simulink model "AutonomousModel_V3"  (R2020b)
settings: Solver=ode23t  StartTime=0.0  StopTime=180.1  FixedStep=0.05  RelTol=1e-3  EnableMultiTasking=on
model workspace (MAT data in the model file):
  mapForSim : object (value not decoded)
  occGrid : robotics.BinaryOccupancyGrid (value not decoded)
undefined symbols (not defined in the file): cellLevel, cellPose, cellTypeArray, FloorSurface, isoPoses, platformPoses, PlowSurface, Ref, RobotSurface, WallSurface, X, Y, Z
libraries: sm_lib x286, nesl_utility x157, simulink x72, pid_lib x3
(part 2 of 14)

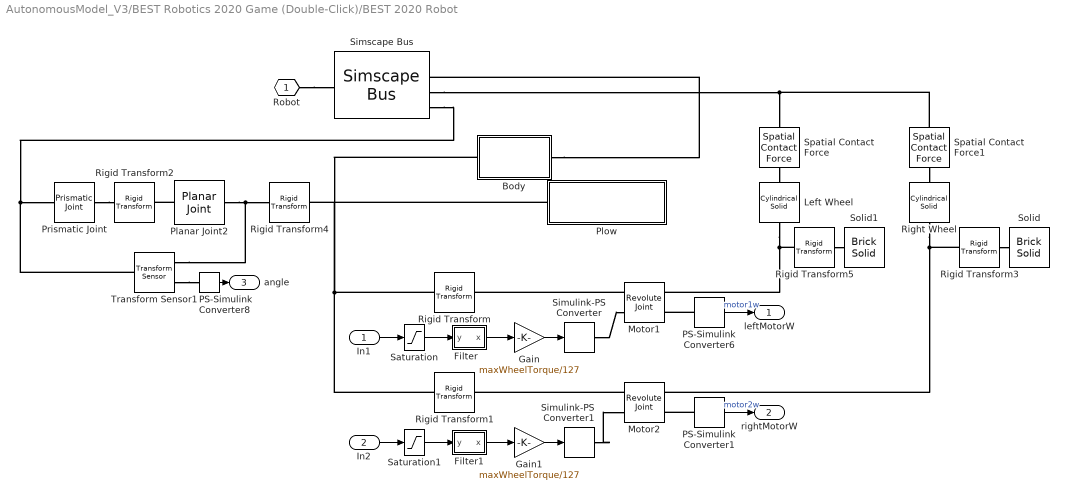
== system AutonomousModel_V3/BEST Robotics 2020 Game (Double-Click)/BEST 2020 Robot ==
  In1 : Inport
  In2 : Inport  Port=2
  Body : Subsystem
  Filter : Subsystem
  Filter1 : Subsystem
  Gain : Gain  Gain=maxWheelTorque/127
  Gain1 : Gain  Gain=maxWheelTorque/127
  Left Wheel : sm_lib/Body Elements/Cylindrical Solid  GraphicAmbientColor=[0.15 0.15 0.15 1.0]  BasedOnType=Mass  CenterOfMass=[0 0 0]  CenterOfMassUnits=m  GraphicDiffuseColor=wheelColor  CylinderLength=wheelThickness  CylinderLengthUnits=m  CylinderRadius=wheelRadius  CylinderRadiusUnits=m  Density=1000  DensityUnits=kg/m^3  DoExposeReferenceFrame=on  GraphicEmissiveColor=[0.0 0.0 0.0 1.0]  ExportEntireGeometry=on  SerializedFrames=<Frames/>  MarkerShape=Sphere  MarkerSize=10  GraphicType=FromGeometry  InertiaType=CalculateFromGeometry  Mass=wheelMass  MassUnits=kg  MomentsOfInertia=[1 1 1]  MomentsOfInertiaUnits=kg*m^2  GraphicOpacity=1.0  ProductsOfInertia=[1 1 1]  ProductsOfInertiaUnits=kg*m^2  GraphicShininess=75  GraphicSpecularColor=[0.5 0.5 0.5 1.0]  GraphicVisPropType=SimpleVisualProperties
  Motor1 : sm_lib/Joints/Revolute Joint  JointMode=Normal  SenseConstraintForce=off  SenseConstraintForceX=off  SenseConstraintForceY=off  SenseConstraintForceZ=off  SenseConstraintTorque=off  SenseConstraintTorqueX=off  SenseConstraintTorqueY=off  SenseConstraintTorqueZ=off  SenseTotalForce=off  SenseTotalForceX=off  SenseTotalForceY=off  SenseTotalForceZ=off  SenseTotalTorque=off  SenseTotalTorqueX=off  SenseTotalTorqueY=off  SenseTotalTorqueZ=off  CompositeWrenchDir=FollowerOnBase  CompositeWrenchFrame=BaseFrame  EquilibriumPosition=0  EquilibriumPositionUnits=deg  SpringStiffness=0  SpringStiffnessUnits=N*m/deg  DampingCoefficient=0.004  DampingCoefficientUnits=N*m/(deg/s)  TorqueActuationMode=InputTorque  MotionActuationMode=ComputedMotion  SensePosition=off  SenseVelocity=on  SenseAcceleration=off  SenseTorqueForce=off  SenseLowerLimitTorqueForce=off  SenseUpperLimitTorqueForce=off  LowerLimitSpecify=off  LowerLimitBound=-90  LowerLimitBoundUnits=deg  LowerLimitStiffness=1e4  LowerLimitStiffnessUnits=N*m/deg  LowerLimitDamping=10  LowerLimitDampingUnits=N*m/(deg/s)  LowerLimitTransitionRegionWidth=0.1  LowerLimitTransitionRegionWidthUnits=deg  UpperLimitSpecify=off  UpperLimitBound=90  UpperLimitBoundUnits=deg  UpperLimitStiffness=1e4  UpperLimitStiffnessUnits=N*m/deg  UpperLimitDamping=10  UpperLimitDampingUnits=N*m/(deg/s)  UpperLimitTransitionRegionWidth=0.1  UpperLimitTransitionRegionWidthUnits=deg  PositionTargetSpecify=off  PositionTargetPriority=High  PositionTargetValue=0  PositionTargetValueUnits=deg  VelocityTargetSpecify=off  VelocityTargetPriority=High  VelocityTargetValue=0  VelocityTargetValueUnits=deg/s
  Motor2 : sm_lib/Joints/Revolute Joint  JointMode=Normal  SenseConstraintForce=off  SenseConstraintForceX=off  SenseConstraintForceY=off  SenseConstraintForceZ=off  SenseConstraintTorque=off  SenseConstraintTorqueX=off  SenseConstraintTorqueY=off  SenseConstraintTorqueZ=off  SenseTotalForce=off  SenseTotalForceX=off  SenseTotalForceY=off  SenseTotalForceZ=off  SenseTotalTorque=off  SenseTotalTorqueX=off  SenseTotalTorqueY=off  SenseTotalTorqueZ=off  CompositeWrenchDir=FollowerOnBase  CompositeWrenchFrame=BaseFrame  EquilibriumPosition=0  EquilibriumPositionUnits=deg  SpringStiffness=0  SpringStiffnessUnits=N*m/deg  DampingCoefficient=0.004  DampingCoefficientUnits=N*m/(deg/s)  TorqueActuationMode=InputTorque  MotionActuationMode=ComputedMotion  SensePosition=off  SenseVelocity=on  SenseAcceleration=off  SenseTorqueForce=off  SenseLowerLimitTorqueForce=off  SenseUpperLimitTorqueForce=off  LowerLimitSpecify=off  LowerLimitBound=-90  LowerLimitBoundUnits=deg  LowerLimitStiffness=1e4  LowerLimitStiffnessUnits=N*m/deg  LowerLimitDamping=10  LowerLimitDampingUnits=N*m/(deg/s)  LowerLimitTransitionRegionWidth=0.1  LowerLimitTransitionRegionWidthUnits=deg  UpperLimitSpecify=off  UpperLimitBound=90  UpperLimitBoundUnits=deg  UpperLimitStiffness=1e4  UpperLimitStiffnessUnits=N*m/deg  UpperLimitDamping=10  UpperLimitDampingUnits=N*m/(deg/s)  UpperLimitTransitionRegionWidth=0.1  UpperLimitTransitionRegionWidthUnits=deg  PositionTargetSpecify=off  PositionTargetPriority=High  PositionTargetValue=0  PositionTargetValueUnits=deg  VelocityTargetSpecify=off  VelocityTargetPriority=High  VelocityTargetValue=0  VelocityTargetValueUnits=deg/s
  PS-Simulink Converter1 : nesl_utility/PS-Simulink Converter  PhysicalDomain=network_engine_domain  SubClassName=ps_output  LeftPortType=input  RightPortType=output  PseudoPeriodic=off  Frequencies=[]  Unit=1  AffineConversion=off
  PS-Simulink Converter6 : nesl_utility/PS-Simulink Converter  PhysicalDomain=network_engine_domain  SubClassName=ps_output  LeftPortType=input  RightPortType=output  PseudoPeriodic=off  Frequencies=[]  Unit=1  AffineConversion=off
  PS-Simulink Converter8 : nesl_utility/PS-Simulink Converter  PhysicalDomain=network_engine_domain  SubClassName=ps_output  LeftPortType=input  RightPortType=output  PseudoPeriodic=off  Frequencies=[]  Unit=deg  AffineConversion=off
  Planar Joint2 : sm_lib/Joints/Planar Joint  JointMode=Normal  SenseConstraintForce=off  SenseConstraintForceX=off  SenseConstraintForceY=off  SenseConstraintForceZ=off  SenseConstraintTorque=off  SenseConstraintTorqueX=off  SenseConstraintTorqueY=off  SenseConstraintTorqueZ=off  SenseTotalForce=off  SenseTotalForceX=off  SenseTotalForceY=off  SenseTotalForceZ=off  SenseTotalTorque=off  SenseTotalTorqueX=off  SenseTotalTorqueY=off  SenseTotalTorqueZ=off  CompositeWrenchDir=FollowerOnBase  CompositeWrenchFrame=BaseFrame  PxEquilibriumPosition=0  PxEquilibriumPositionUnits=m  PxSpringStiffness=0  PxSpringStiffnessUnits=N/m  PxDampingCoefficient=0  PxDampingCoefficientUnits=N/(m/s)  PxTorqueActuationMode=NoTorque  PxMotionActuationMode=ComputedMotion  PxSensePosition=off  PxSenseVelocity=off  PxSenseAcceleration=off  PxSenseTorqueForce=off  PxSenseLowerLimitTorqueForce=off  PxSenseUpperLimitTorqueForce=off  PxLowerLimitSpecify=off  PxLowerLimitBound=-1  PxLowerLimitBoundUnits=m  PxLowerLimitStiffness=1e6  PxLowerLimitStiffnessUnits=N/m  PxLowerLimitDamping=1e3  PxLowerLimitDampingUnits=N/(m/s)  PxLowerLimitTransitionRegionWidth=1e-4  PxLowerLimitTransitionRegionWidthUnits=m  PxUpperLimitSpecify=off  PxUpperLimitBound=1  PxUpperLimitBoundUnits=m  PxUpperLimitStiffness=1e6  PxUpperLimitStiffnessUnits=N/m  PxUpperLimitDamping=1e3  PxUpperLimitDampingUnits=N/(m/s)  PxUpperLimitTransitionRegionWidth=1e-4  PxUpperLimitTransitionRegionWidthUnits=m  PxPositionTargetSpecify=on  PxPositionTargetPriority=High  PxPositionTargetValue=startPose(1)  PxPositionTargetValueUnits=m  PxVelocityTargetSpecify=off  PxVelocityTargetPriority=High  PxVelocityTargetValue=0  PxVelocityTargetValueUnits=m/s  PyEquilibriumPosition=0  PyEquilibriumPositionUnits=m  PySpringStiffness=0  PySpringStiffnessUnits=N/m  PyDampingCoefficient=0  PyDampingCoefficientUnits=N/(m/s)  PyTorqueActuationMode=NoTorque  PyMotionActuationMode=ComputedMotion  PySensePosition=off  PySenseVelocity=off  PySenseAcceleration=off  PySenseTorqueForce=off  PySenseLowerLimitTorqueForce=off  PySenseUpperLimitTorqueForce=off  PyLowerLimitSpecify=off  PyLowerLimitBound=-1  PyLowerLimitBoundUnits=m  PyLowerLimitStiffness=1e6  PyLowerLimitStiffnessUnits=N/m  PyLowerLimitDamping=1e3  PyLowerLimitDampingUnits=N/(m/s)  PyLowerLimitTransitionRegionWidth=1e-4  PyLowerLimitTransitionRegionWidthUnits=m  PyUpperLimitSpecify=off  PyUpperLimitBound=1  PyUpperLimitBoundUnits=m  PyUpperLimitStiffness=1e6  PyUpperLimitStiffnessUnits=N/m  PyUpperLimitDamping=1e3  PyUpperLimitDampingUnits=N/(m/s)  PyUpperLimitTransitionRegionWidth=1e-4  PyUpperLimitTransitionRegionWidthUnits=m  PyPositionTargetSpecify=on  PyPositionTargetPriority=High  PyPositionTargetValue=startPose(2)  PyPositionTargetValueUnits=m  PyVelocityTargetSpecify=off  PyVelocityTargetPriority=High  PyVelocityTargetValue=0  PyVelocityTargetValueUnits=m/s  RzEquilibriumPosition=0  RzEquilibriumPositionUnits=deg  RzSpringStiffness=0  RzSpringStiffnessUnits=N*m/deg  RzDampingCoefficient=0  RzDampingCoefficientUnits=N*m/(deg/s)  RzTorqueActuationMode=NoTorque  RzMotionActuationMode=ComputedMotion  RzSensePosition=off  RzSenseVelocity=off  RzSenseAcceleration=off  RzSenseTorqueForce=off  RzSenseLowerLimitTorqueForce=off  RzSenseUpperLimitTorqueForce=off  RzLowerLimitSpecify=off  RzLowerLimitBound=-90  RzLowerLimitBoundUnits=deg  RzLowerLimitStiffness=1e4  RzLowerLimitStiffnessUnits=N*m/deg  RzLowerLimitDamping=10  RzLowerLimitDampingUnits=N*m/(deg/s)  RzLowerLimitTransitionRegionWidth=0.1  RzLowerLimitTransitionRegionWidthUnits=deg  RzUpperLimitSpecify=off  RzUpperLimitBound=90  RzUpperLimitBoundUnits=deg  RzUpperLimitStiffness=1e4  RzUpperLimitStiffnessUnits=N*m/deg  RzUpperLimitDamping=10  RzUpperLimitDampingUnits=N*m/(deg/s)  RzUpperLimitTransitionRegionWidth=0.1  RzUpperLimitTransitionRegionWidthUnits=deg  RzPositionTargetSpecify=off  RzPositionTargetPriority=High  RzPositionTargetValue=0  RzPositionTargetValueUnits=deg  RzVelocityTargetSpecify=off  RzVelocityTargetPriority=High  RzVelocityTargetValue=0  RzVelocityTargetValueUnits=deg/s
  Plow : Subsystem
  Prismatic Joint : sm_lib/Joints/Prismatic Joint  JointMode=Normal  SenseConstraintForce=off  SenseConstraintForceX=off  SenseConstraintForceY=off  SenseConstraintForceZ=off  SenseConstraintTorque=off  SenseConstraintTorqueX=off  SenseConstraintTorqueY=off  SenseConstraintTorqueZ=off  SenseTotalForce=off  SenseTotalForceX=off  SenseTotalForceY=off  SenseTotalForceZ=off  SenseTotalTorque=off  SenseTotalTorqueX=off  SenseTotalTorqueY=off  SenseTotalTorqueZ=off  CompositeWrenchDir=FollowerOnBase  CompositeWrenchFrame=BaseFrame  EquilibriumPosition=0  EquilibriumPositionUnits=m  SpringStiffness=0  SpringStiffnessUnits=N/m  DampingCoefficient=0  DampingCoefficientUnits=N/(m/s)  TorqueActuationMode=NoTorque  MotionActuationMode=ComputedMotion  SensePosition=off  SenseVelocity=off  SenseAcceleration=off  SenseTorqueForce=off  SenseLowerLimitTorqueForce=off  SenseUpperLimitTorqueForce=off  LowerLimitSpecify=off  LowerLimitBound=-1  LowerLimitBoundUnits=m  LowerLimitStiffness=1e6  LowerLimitStiffnessUnits=N/m  LowerLimitDamping=1e3  LowerLimitDampingUnits=N/(m/s)  LowerLimitTransitionRegionWidth=1e-4  LowerLimitTransitionRegionWidthUnits=m  UpperLimitSpecify=off  UpperLimitBound=1  UpperLimitBoundUnits=m  UpperLimitStiffness=1e6  UpperLimitStiffnessUnits=N/m  UpperLimitDamping=1e3  UpperLimitDampingUnits=N/(m/s)  UpperLimitTransitionRegionWidth=1e-4  UpperLimitTransitionRegionWidthUnits=m  PositionTargetSpecify=on  PositionTargetPriority=High  PositionTargetValue=0.02  PositionTargetValueUnits=m  VelocityTargetSpecify=off  VelocityTargetPriority=High  VelocityTargetValue=0  VelocityTargetValueUnits=m/s
  Right Wheel : sm_lib/Body Elements/Cylindrical Solid  GraphicAmbientColor=[0.15 0.15 0.15 1.0]  BasedOnType=Mass  CenterOfMass=[0 0 0]  CenterOfMassUnits=m  GraphicDiffuseColor=wheelColor  CylinderLength=wheelThickness  CylinderLengthUnits=m  CylinderRadius=wheelRadius  CylinderRadiusUnits=m  Density=1000  DensityUnits=kg/m^3  DoExposeReferenceFrame=on  GraphicEmissiveColor=[0.0 0.0 0.0 1.0]  ExportEntireGeometry=on  SerializedFrames=<Frames/>  MarkerShape=Sphere  MarkerSize=10  GraphicType=FromGeometry  InertiaType=CalculateFromGeometry  Mass=wheelMass  MassUnits=kg  MomentsOfInertia=[1 1 1]  MomentsOfInertiaUnits=kg*m^2  GraphicOpacity=1.0  ProductsOfInertia=[1 1 1]  ProductsOfInertiaUnits=kg*m^2  GraphicShininess=75  GraphicSpecularColor=[0.5 0.5 0.5 1.0]  GraphicVisPropType=SimpleVisualProperties
  Rigid Transform : sm_lib/Frames and Transforms/Rigid Transform  TranslationMethod=StandardAxis  TranslationStandardOffset=wheelBase/2  TranslationLengthUnit=m  TranslationStandardAxis=+Y  TranslationCartesianOffset=[0 0 0]  TranslationROffset=0  TranslationROffsetUnits=m  TranslationZOffset=0  TranslationZOffsetUnits=m  TranslationThetaOffset=0  TranslationThetaOffsetUnits=deg  RotationMethod=AlignedAxes  RotationAngleUnits=deg  RotationStandardAxis=+Z  RotationAngle=0.0  RotationArbitraryAxis=[0 0 1]  FollAlignAxisA=+Z  BaseAlignAxisA=+Y  FollAlignAxisB=+X  BaseAlignAxisB=+X  RotationSequenceAxes=FollowerAxes  RotationSequence=XYX  RotationSequenceAngles=[0 0 0]  RotationSequenceAnglesUnits=deg  RotationMatrix=[1 0 0; 0 1 0; 0 0 1]
  Rigid Transform1 : sm_lib/Frames and Transforms/Rigid Transform  TranslationMethod=StandardAxis  TranslationStandardOffset=wheelBase/2  TranslationLengthUnit=m  TranslationStandardAxis=-Y  TranslationCartesianOffset=[0 0 0]  TranslationROffset=0  TranslationROffsetUnits=m  TranslationZOffset=0  TranslationZOffsetUnits=m  TranslationThetaOffset=0  TranslationThetaOffsetUnits=deg  RotationMethod=AlignedAxes  RotationAngleUnits=deg  RotationStandardAxis=+Z  RotationAngle=0.0  RotationArbitraryAxis=[0 0 1]  FollAlignAxisA=+Z  BaseAlignAxisA=+Y  FollAlignAxisB=+X  BaseAlignAxisB=+X  RotationSequenceAxes=FollowerAxes  RotationSequence=XYX  RotationSequenceAngles=[0 0 0]  RotationSequenceAnglesUnits=deg  RotationMatrix=[1 0 0; 0 1 0; 0 0 1]
  Rigid Transform2 : sm_lib/Frames and Transforms/Rigid Transform  TranslationMethod=StandardAxis  TranslationStandardOffset=wheelRadius  TranslationLengthUnit=m  TranslationStandardAxis=+Z  TranslationCartesianOffset=[0 0 0]  TranslationROffset=0  TranslationROffsetUnits=m  TranslationZOffset=0  TranslationZOffsetUnits=m  TranslationThetaOffset=0  TranslationThetaOffsetUnits=deg  RotationMethod=None  RotationAngleUnits=deg  RotationStandardAxis=+Z  RotationAngle=0.0  RotationArbitraryAxis=[0 0 1]  FollAlignAxisA=+Z  BaseAlignAxisA=+Y  FollAlignAxisB=+X  BaseAlignAxisB=+X  RotationSequenceAxes=FollowerAxes  RotationSequence=XYX  RotationSequenceAngles=[0 0 0]  RotationSequenceAnglesUnits=deg  RotationMatrix=[1 0 0; 0 1 0; 0 0 1]
  Rigid Transform3 : sm_lib/Frames and Transforms/Rigid Transform  TranslationMethod=Cartesian  TranslationStandardOffset=0  TranslationLengthUnit=m  TranslationStandardAxis=+Z  TranslationCartesianOffset=[wheelRadius/2 0 0]  TranslationROffset=0  TranslationROffsetUnits=m  TranslationZOffset=0  TranslationZOffsetUnits=m  TranslationThetaOffset=0  TranslationThetaOffsetUnits=deg  RotationMethod=None  RotationAngleUnits=deg  RotationStandardAxis=+Z  RotationAngle=0.0  RotationArbitraryAxis=[0 0 1]  FollAlignAxisA=+X  BaseAlignAxisA=+Y  FollAlignAxisB=+Y  BaseAlignAxisB=+Z  RotationSequenceAxes=FollowerAxes  RotationSequence=XYX  RotationSequenceAngles=[0 0 0]  RotationSequenceAnglesUnits=deg  RotationMatrix=[1 0 0; 0 1 0; 0 0 1]
  Rigid Transform4 : sm_lib/Frames and Transforms/Rigid Transform  TranslationMethod=None  TranslationStandardOffset=0  TranslationLengthUnit=m  TranslationStandardAxis=+Z  TranslationCartesianOffset=[0 0 0]  TranslationROffset=0  TranslationROffsetUnits=m  TranslationZOffset=0  TranslationZOffsetUnits=m  TranslationThetaOffset=0  TranslationThetaOffsetUnits=deg  RotationMethod=StandardAxis  RotationAngleUnits=deg  RotationStandardAxis=+Z  RotationAngle=180*choice  RotationArbitraryAxis=[0 0 1]  FollAlignAxisA=+X  BaseAlignAxisA=+Y  FollAlignAxisB=+Y  BaseAlignAxisB=+Z  RotationSequenceAxes=FollowerAxes  RotationSequence=XYX  RotationSequenceAngles=[0 0 0]  RotationSequenceAnglesUnits=deg  RotationMatrix=[1 0 0; 0 1 0; 0 0 1]
  Rigid Transform5 : sm_lib/Frames and Transforms/Rigid Transform  TranslationMethod=Cartesian  TranslationStandardOffset=0  TranslationLengthUnit=m  TranslationStandardAxis=+Z  TranslationCartesianOffset=[wheelRadius/2 0 0]  TranslationROffset=0  TranslationROffsetUnits=m  TranslationZOffset=0  TranslationZOffsetUnits=m  TranslationThetaOffset=0  TranslationThetaOffsetUnits=deg  RotationMethod=None  RotationAngleUnits=deg  RotationStandardAxis=+Z  RotationAngle=0.0  RotationArbitraryAxis=[0 0 1]  FollAlignAxisA=+X  BaseAlignAxisA=+Y  FollAlignAxisB=+Y  BaseAlignAxisB=+Z  RotationSequenceAxes=FollowerAxes  RotationSequence=XYX  RotationSequenceAngles=[0 0 0]  RotationSequenceAnglesUnits=deg  RotationMatrix=[1 0 0; 0 1 0; 0 0 1]
  Saturation : Saturate  UpperLimit=127  LowerLimit=-127  ZeroCross=off
  Saturation1 : Saturate  UpperLimit=127  LowerLimit=-127  ZeroCross=off
  Simscape Bus : SimscapeBus  HierarchyStrings=PlowSurface;RobotSurface;FloorSurface;Ref
  Simulink-PS Converter : nesl_utility/Simulink-PS Converter  PhysicalDomain=network_engine_domain  SubClassName=ps_input  LeftPortType=input  RightPortType=output  PseudoPeriodic=off  Frequencies=[]  NoiseDistribution=none  NoiseParameters=[]  Unit=1  AffineConversion=off  FilteringAndDerivatives=provide  SimscapeFilterOrder=1  InputFilterTimeConstant=0.05  UdotUserProvided=0
  Simulink-PS Converter1 : nesl_utility/Simulink-PS Converter  PhysicalDomain=network_engine_domain  SubClassName=ps_input  LeftPortType=input  RightPortType=output  PseudoPeriodic=off  Frequencies=[]  NoiseDistribution=none  NoiseParameters=[]  Unit=1  AffineConversion=off  FilteringAndDerivatives=provide  SimscapeFilterOrder=1  InputFilterTimeConstant=0.05  UdotUserProvided=0
  Solid : sm_lib/Body Elements/Brick Solid  GraphicAmbientColor=[0.15 0.15 0.15 1.0]  BasedOnType=Density  BrickDimensions=[wheelRadius*0.8 wheelThickness*1.05 wheelThickness*1.05]  BrickDimensionUnits=m  CenterOfMass=[0 0 0]  CenterOfMassUnits=m  GraphicDiffuseColor=[0.0 0.8 0.8]  Density=1000  DensityUnits=kg/m^3  DoExposeReferenceFrame=on  GraphicEmissiveColor=[0.0 0.0 0.0 1.0]  ExportEntireGeometry=off  SerializedFrames=<Frames/>  MarkerShape=Sphere  MarkerSize=10  GraphicType=FromGeometry  InertiaType=PointMass  Mass=0.001  MassUnits=kg  MomentsOfInertia=[1 1 1]  MomentsOfInertiaUnits=kg*m^2  GraphicOpacity=1.0  ProductsOfInertia=[1 1 1]  ProductsOfInertiaUnits=kg*m^2  GraphicShininess=75  GraphicSpecularColor=[0.5 0.5 0.5 1.0]  GraphicVisPropType=SimpleVisualProperties
  Solid1 : sm_lib/Body Elements/Brick Solid  GraphicAmbientColor=[0.15 0.15 0.15 1.0]  BasedOnType=Density  BrickDimensions=[wheelRadius*0.8 wheelThickness*1.05 wheelThickness*1.05]  BrickDimensionUnits=m  CenterOfMass=[0 0 0]  CenterOfMassUnits=m  GraphicDiffuseColor=[0.0 0.8 0.8]  Density=1000  DensityUnits=kg/m^3  DoExposeReferenceFrame=on  GraphicEmissiveColor=[0.0 0.0 0.0 1.0]  ExportEntireGeometry=off  SerializedFrames=<Frames/>  MarkerShape=Sphere  MarkerSize=10  GraphicType=FromGeometry  InertiaType=PointMass  Mass=0.001  MassUnits=kg  MomentsOfInertia=[1 1 1]  MomentsOfInertiaUnits=kg*m^2  GraphicOpacity=1.0  ProductsOfInertia=[1 1 1]  ProductsOfInertiaUnits=kg*m^2  GraphicShininess=75  GraphicSpecularColor=[0.5 0.5 0.5 1.0]  GraphicVisPropType=SimpleVisualProperties
  Spatial Contact Force : sm_lib/Forces and Torques/Spatial Contact Force  CoefficientOfDynamicFriction=0.5  CoefficientOfStaticFriction=0.7  NormalDamping=1e2  NormalDampingUnits=N/(m/s)  NormalStiffness=1e4  NormalStiffnessUnits=N/m  FrictionalCriticalVelocity=1e-3  FrictionalCriticalVelocityUnits=m/s  ZeroCrossDetectContactStartAndEnd=off  SenseFrictionalForceMagnitude=off  SenseNormalForceMagnitude=off  SenseSeparationDistance=off  NormalTransitionRegionWidth=1e-2  NormalTransitionRegionWidthUnits=m  FrictionType=SmoothStickSlip
  Spatial Contact Force1 : sm_lib/Forces and Torques/Spatial Contact Force  CoefficientOfDynamicFriction=0.5  CoefficientOfStaticFriction=0.7  NormalDamping=1e2  NormalDampingUnits=N/(m/s)  NormalStiffness=1e4  NormalStiffnessUnits=N/m  FrictionalCriticalVelocity=1e-3  FrictionalCriticalVelocityUnits=m/s  ZeroCrossDetectContactStartAndEnd=off  SenseFrictionalForceMagnitude=off  SenseNormalForceMagnitude=off  SenseSeparationDistance=off  NormalTransitionRegionWidth=1e-2  NormalTransitionRegionWidthUnits=m  FrictionType=SmoothStickSlip
  Transform Sensor1 : sm_lib/Frames and Transforms/Transform Sensor  MeasurementFrame=World  SenseAngle=on  SenseAxis=off  SenseAngle1=off  SenseAngle2=off  SenseAngle3=off  SenseQ=off  SenseR=off  SenseOmegaX=off  SenseOmegaY=off  SenseOmegaZ=off  SenseOmega1=off  SenseOmega2=off  SenseOmega3=off  SenseQDot=off  SenseRDot=off  SenseAlphaX=off  SenseAlphaY=off  SenseAlphaZ=off  SenseAlpha1=off  SenseAlpha2=off  SenseAlpha3=off  SenseQDDot=off  SenseRDDot=off  SenseX=off  SenseY=off  SenseZ=off  SenseRad=off  SenseAzim=off  SenseDist=off  SenseInc=off  SenseXDot=off  SenseYDot=off  SenseZDot=off  SenseRadDot=off  SenseAzimDot=off  SenseDistDot=off  SenseIncDot=off  SenseXDDot=off  SenseYDDot=off  SenseZDDot=off  SenseRadDDot=off  SenseAzimDDot=off  SenseDistDDot=off  SenseIncDDot=off
  Robot : PMIOPort  Side=Right
  leftMotorW : Outport
  rightMotorW : Outport  Port=2
  angle : Outport  Port=3
  wires:
  PS-Simulink Converter6/1 -> leftMotorW/1  "motor1w"
  PS-Simulink Converter1/1 -> rightMotorW/1  "motor2w"
  Filter1/1(x) -> Gain1/1
  Filter/1(x) -> Gain/1
  Gain/1 -> Simulink-PS Converter/1
  Gain1/1 -> Simulink-PS Converter1/1
  In1/1 -> Saturation/1
  In2/1 -> Saturation1/1
  PS-Simulink Converter8/1 -> angle/1
  Saturation/1 -> Filter/1(y)
  Saturation1/1 -> Filter1/1(y)
  connections:
  PS-Simulink Converter1/LConn1 -- Motor2/RConn2
  PS-Simulink Converter6/LConn1 -- Motor1/RConn2
  Simulink-PS Converter/RConn1 -- Motor1/LConn2
  Simulink-PS Converter1/RConn1 -- Motor2/LConn2
  Right Wheel/RConn1 -- Rigid Transform3/LConn1 -- Motor2/RConn1
  Motor1/LConn1 -- Rigid Transform/RConn1
  Planar Joint2/LConn1 -- Rigid Transform2/RConn1
  Simscape Bus/LConn4 -- Transform Sensor1/LConn1 -- Prismatic Joint/LConn1
  Motor2/LConn1 -- Rigid Transform1/RConn1
  Rigid Transform5/LConn1 -- Left Wheel/RConn1 -- Motor1/RConn1
  Rigid Transform/LConn1 -- Rigid Transform1/LConn1 -- Body/LConn1 -- Rigid Transform4/RConn1 -- Plow/LConn1
  Planar Joint2/RConn1 -- Rigid Transform4/LConn1 -- Transform Sensor1/RConn1
  Prismatic Joint/RConn1 -- Rigid Transform2/LConn1
  Transform Sensor1/RConn2 -- PS-Simulink Converter8/LConn1
  Robot/RConn1 -- Simscape Bus/RConn1
  Rigid Transform3/RConn1 -- Solid/RConn1
  Rigid Transform5/RConn1 -- Solid1/RConn1
  Spatial Contact Force/RConn1 -- Left Wheel/LConn1
  Spatial Contact Force1/RConn1 -- Right Wheel/LConn1
  Simscape Bus/LConn3 -- Spatial Contact Force1/LConn1 -- Spatial Contact Force/LConn1
  Body/RConn1 -- Simscape Bus/LConn2

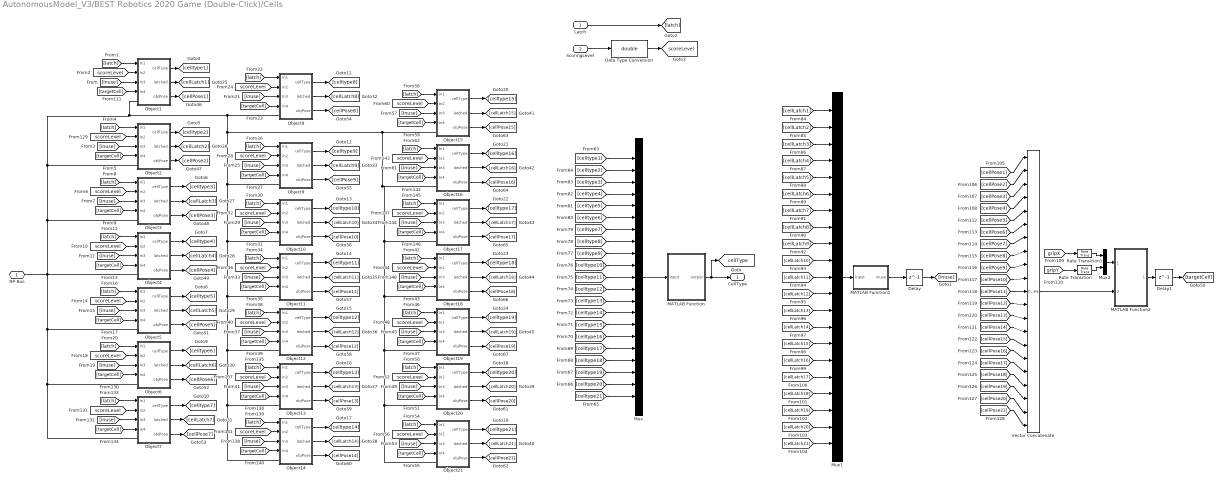
== system AutonomousModel_V3/BEST Robotics 2020 Game (Double-Click)/Cells ==
  Latch : Inport
  ScoringLevel : Inport  Port=2
  Data Type Conversion : DataTypeConversion  OutDataTypeStr=double
  Delay : Delay  DelayLength=1
  Delay1 : Delay  DelayLength=1
  MATLAB Function : MATLAB Function  TreatAsAtomicUnit=on
  MATLAB Function1 : MATLAB Function  TreatAsAtomicUnit=on
  MATLAB Function2 : MATLAB Function  TreatAsAtomicUnit=on
  Mux : Mux  Inputs=21
  Mux1 : Mux  Inputs=21
  Mux2 : Mux  Inputs=2
  Object1 : Subsystem  mask(RP Rectangle-Disc obstacle){objId=1}
      mask prompts: objId "Id"
      mask help: This block introduces a rectangle obstacle to the virtual environment. The obstacle dynamics include exerting the necessary contact forces with the robots as well as detectability by the ultrasonic sensor when used in a MathWorks provided virtual environment.
      mask init:
      | id=get_param(gcb,'objId');
      | 
      | set_param([gcb, '/Goto'],'GotoTag',['objInfo' num2str(id)])
      mask TypeOptions objId: MATLAB Function/objId
  Object10 : Subsystem  mask(RP Rectangle-Disc obstacle){objId=10}
      mask prompts: objId "Id"
      mask help: This block introduces a rectangle obstacle to the virtual environment. The obstacle dynamics include exerting the necessary contact forces with the robots as well as detectability by the ultrasonic sensor when used in a MathWorks provided virtual environment.
      mask init:
      | id=get_param(gcb,'objId');
      | 
      | set_param([gcb, '/Goto'],'GotoTag',['objInfo' num2str(id)])
      mask TypeOptions objId: MATLAB Function/objId
  Object11 : Subsystem  mask(RP Rectangle-Disc obstacle){objId=11}
      mask prompts: objId "Id"
      mask help: This block introduces a rectangle obstacle to the virtual environment. The obstacle dynamics include exerting the necessary contact forces with the robots as well as detectability by the ultrasonic sensor when used in a MathWorks provided virtual environment.
      mask init:
      | id=get_param(gcb,'objId');
      | 
      | set_param([gcb, '/Goto'],'GotoTag',['objInfo' num2str(id)])
      mask TypeOptions objId: MATLAB Function/objId
  Object12 : Subsystem  mask(RP Rectangle-Disc obstacle){objId=12}
      mask prompts: objId "Id"
      mask help: This block introduces a rectangle obstacle to the virtual environment. The obstacle dynamics include exerting the necessary contact forces with the robots as well as detectability by the ultrasonic sensor when used in a MathWorks provided virtual environment.
      mask init:
      | id=get_param(gcb,'objId');
      | 
      | set_param([gcb, '/Goto'],'GotoTag',['objInfo' num2str(id)])
      mask TypeOptions objId: MATLAB Function/objId
  Object13 : Subsystem  mask(RP Rectangle-Disc obstacle){objId=13}
      mask prompts: objId "Id"
      mask help: This block introduces a rectangle obstacle to the virtual environment. The obstacle dynamics include exerting the necessary contact forces with the robots as well as detectability by the ultrasonic sensor when used in a MathWorks provided virtual environment.
      mask init:
      | id=get_param(gcb,'objId');
      | 
      | set_param([gcb, '/Goto'],'GotoTag',['objInfo' num2str(id)])
      mask TypeOptions objId: MATLAB Function/objId
  Object14 : Subsystem  mask(RP Rectangle-Disc obstacle){objId=14}
      mask prompts: objId "Id"
      mask help: This block introduces a rectangle obstacle to the virtual environment. The obstacle dynamics include exerting the necessary contact forces with the robots as well as detectability by the ultrasonic sensor when used in a MathWorks provided virtual environment.
      mask init:
      | id=get_param(gcb,'objId');
      | 
      | set_param([gcb, '/Goto'],'GotoTag',['objInfo' num2str(id)])
      mask TypeOptions objId: MATLAB Function/objId
  Object15 : Subsystem  mask(RP Rectangle-Disc obstacle){objId=15}
      mask prompts: objId "Id"
      mask help: This block introduces a rectangle obstacle to the virtual environment. The obstacle dynamics include exerting the necessary contact forces with the robots as well as detectability by the ultrasonic sensor when used in a MathWorks provided virtual environment.
      mask init:
      | id=get_param(gcb,'objId');
      | 
      | set_param([gcb, '/Goto'],'GotoTag',['objInfo' num2str(id)])
      mask TypeOptions objId: MATLAB Function/objId
  Object16 : Subsystem  mask(RP Rectangle-Disc obstacle){objId=16}
      mask prompts: objId "Id"
      mask help: This block introduces a rectangle obstacle to the virtual environment. The obstacle dynamics include exerting the necessary contact forces with the robots as well as detectability by the ultrasonic sensor when used in a MathWorks provided virtual environment.
      mask init:
      | id=get_param(gcb,'objId');
      | 
      | set_param([gcb, '/Goto'],'GotoTag',['objInfo' num2str(id)])
      mask TypeOptions objId: MATLAB Function/objId
  Object17 : Subsystem  mask(RP Rectangle-Disc obstacle){objId=17}
      mask prompts: objId "Id"
      mask help: This block introduces a rectangle obstacle to the virtual environment. The obstacle dynamics include exerting the necessary contact forces with the robots as well as detectability by the ultrasonic sensor when used in a MathWorks provided virtual environment.
      mask init:
      | id=get_param(gcb,'objId');
      | 
      | set_param([gcb, '/Goto'],'GotoTag',['objInfo' num2str(id)])
      mask TypeOptions objId: MATLAB Function/objId
  Object18 : Subsystem  mask(RP Rectangle-Disc obstacle){objId=18}
      mask prompts: objId "Id"
      mask help: This block introduces a rectangle obstacle to the virtual environment. The obstacle dynamics include exerting the necessary contact forces with the robots as well as detectability by the ultrasonic sensor when used in a MathWorks provided virtual environment.
      mask init:
      | id=get_param(gcb,'objId');
      | 
      | set_param([gcb, '/Goto'],'GotoTag',['objInfo' num2str(id)])
      mask TypeOptions objId: MATLAB Function/objId
  Object19 : Subsystem  mask(RP Rectangle-Disc obstacle){objId=19}
      mask prompts: objId "Id"
      mask help: This block introduces a rectangle obstacle to the virtual environment. The obstacle dynamics include exerting the necessary contact forces with the robots as well as detectability by the ultrasonic sensor when used in a MathWorks provided virtual environment.
      mask init:
      | id=get_param(gcb,'objId');
      | 
      | set_param([gcb, '/Goto'],'GotoTag',['objInfo' num2str(id)])
      mask TypeOptions objId: MATLAB Function/objId
  Object2 : Subsystem  mask(RP Rectangle-Disc obstacle){objId=2}
      mask prompts: objId "Id"
      mask help: This block introduces a rectangle obstacle to the virtual environment. The obstacle dynamics include exerting the necessary contact forces with the robots as well as detectability by the ultrasonic sensor when used in a MathWorks provided virtual environment.
      mask init:
      | id=get_param(gcb,'objId');
      | 
      | set_param([gcb, '/Goto'],'GotoTag',['objInfo' num2str(id)])
      mask TypeOptions objId: MATLAB Function/objId
  Object20 : Subsystem  mask(RP Rectangle-Disc obstacle){objId=20}
      mask prompts: objId "Id"
      mask help: This block introduces a rectangle obstacle to the virtual environment. The obstacle dynamics include exerting the necessary contact forces with the robots as well as detectability by the ultrasonic sensor when used in a MathWorks provided virtual environment.
      mask init:
      | id=get_param(gcb,'objId');
      | 
      | set_param([gcb, '/Goto'],'GotoTag',['objInfo' num2str(id)])
      mask TypeOptions objId: MATLAB Function/objId
  Object21 : Subsystem  mask(RP Rectangle-Disc obstacle){objId=21}
      mask prompts: objId "Id"
      mask help: This block introduces a rectangle obstacle to the virtual environment. The obstacle dynamics include exerting the necessary contact forces with the robots as well as detectability by the ultrasonic sensor when used in a MathWorks provided virtual environment.
      mask init:
      | id=get_param(gcb,'objId');
      | 
      | set_param([gcb, '/Goto'],'GotoTag',['objInfo' num2str(id)])
      mask TypeOptions objId: MATLAB Function/objId
  Object3 : Subsystem  mask(RP Rectangle-Disc obstacle){objId=3}
      mask prompts: objId "Id"
      mask help: This block introduces a rectangle obstacle to the virtual environment. The obstacle dynamics include exerting the necessary contact forces with the robots as well as detectability by the ultrasonic sensor when used in a MathWorks provided virtual environment.
      mask init:
      | id=get_param(gcb,'objId');
      | 
      | set_param([gcb, '/Goto'],'GotoTag',['objInfo' num2str(id)])
      mask TypeOptions objId: MATLAB Function/objId
  Object4 : Subsystem  mask(RP Rectangle-Disc obstacle){objId=4}
      mask prompts: objId "Id"
      mask help: This block introduces a rectangle obstacle to the virtual environment. The obstacle dynamics include exerting the necessary contact forces with the robots as well as detectability by the ultrasonic sensor when used in a MathWorks provided virtual environment.
      mask init:
      | id=get_param(gcb,'objId');
      | 
      | set_param([gcb, '/Goto'],'GotoTag',['objInfo' num2str(id)])
      mask TypeOptions objId: MATLAB Function/objId
  Object5 : Subsystem  mask(RP Rectangle-Disc obstacle){objId=5}
      mask prompts: objId "Id"
      mask help: This block introduces a rectangle obstacle to the virtual environment. The obstacle dynamics include exerting the necessary contact forces with the robots as well as detectability by the ultrasonic sensor when used in a MathWorks provided virtual environment.
      mask init:
      | id=get_param(gcb,'objId');
      | 
      | set_param([gcb, '/Goto'],'GotoTag',['objInfo' num2str(id)])
      mask TypeOptions objId: MATLAB Function/objId
  Object6 : Subsystem  mask(RP Rectangle-Disc obstacle){objId=6}
      mask prompts: objId "Id"
      mask help: This block introduces a rectangle obstacle to the virtual environment. The obstacle dynamics include exerting the necessary contact forces with the robots as well as detectability by the ultrasonic sensor when used in a MathWorks provided virtual environment.
      mask init:
      | id=get_param(gcb,'objId');
      | 
      | set_param([gcb, '/Goto'],'GotoTag',['objInfo' num2str(id)])
      mask TypeOptions objId: MATLAB Function/objId
  Object7 : Subsystem  mask(RP Rectangle-Disc obstacle){objId=7}
      mask prompts: objId "Id"
      mask help: This block introduces a rectangle obstacle to the virtual environment. The obstacle dynamics include exerting the necessary contact forces with the robots as well as detectability by the ultrasonic sensor when used in a MathWorks provided virtual environment.
      mask init:
      | id=get_param(gcb,'objId');
      | 
      | set_param([gcb, '/Goto'],'GotoTag',['objInfo' num2str(id)])
      mask TypeOptions objId: MATLAB Function/objId
  Object8 : Subsystem  mask(RP Rectangle-Disc obstacle){objId=8}
      mask prompts: objId "Id"
      mask help: This block introduces a rectangle obstacle to the virtual environment. The obstacle dynamics include exerting the necessary contact forces with the robots as well as detectability by the ultrasonic sensor when used in a MathWorks provided virtual environment.
      mask init:
      | id=get_param(gcb,'objId');
      | 
      | set_param([gcb, '/Goto'],'GotoTag',['objInfo' num2str(id)])
      mask TypeOptions objId: MATLAB Function/objId
  Object9 : Subsystem  mask(RP Rectangle-Disc obstacle){objId=9}
      mask prompts: objId "Id"
      mask help: This block introduces a rectangle obstacle to the virtual environment. The obstacle dynamics include exerting the necessary contact forces with the robots as well as detectability by the ultrasonic sensor when used in a MathWorks provided virtual environment.
      mask init:
      | id=get_param(gcb,'objId');
      | 
      | set_param([gcb, '/Goto'],'GotoTag',['objInfo' num2str(id)])
      mask TypeOptions objId: MATLAB Function/objId
  Rate Transition : RateTransition
  Rate Transition1 : RateTransition
  Vector Concatenate : Concatenate  NumInputs=21  Mode=Multidimensional array
  RP-Bus : PMIOPort  Side=Left
  CellType : Outport
  tag scope: cellType=global, scoreLevel=global
  wires:
  Mux/1 -> MATLAB Function/1(input)
  MATLAB Function/1(output) -> CellType/1, [cellType]
  MATLAB Function1/1(inuse) -> Delay/1
  Delay/1 -> [inuse]
  Latch/1 -> [latch]
  ScoringLevel/1 -> Data Type Conversion/1
  [inuse] -> Object1/3(In3)
  [scoreLevel] -> Object1/2(In2)
  [latch] -> Object1/1(In1)
  Mux1/1 -> MATLAB Function1/1(input)
  [celltype1] -> Mux/1
  [celltype2] -> Mux/2
  Object1/1(cellType) -> [celltype1]
  Object2/1(cellType) -> [celltype2]
  [celltype3] -> Mux/3
  [celltype4] -> Mux/4
  [celltype5] -> Mux/5
  [celltype6] -> Mux/6
  [celltype7] -> Mux/7
  [celltype8] -> Mux/8
  [celltype9] -> Mux/9
  [celltype10] -> Mux/10
  [celltype11] -> Mux/11
  [celltype12] -> Mux/12
  [celltype13] -> Mux/13
  [celltype14] -> Mux/14
  [celltype15] -> Mux/15
  [celltype16] -> Mux/16
  [celltype17] -> Mux/17
  [celltype18] -> Mux/18
  [celltype19] -> Mux/19
  [celltype20] -> Mux/20
  [celltype21] -> Mux/21
  Object1/2(latched) -> [cellLatch1]
  Object2/2(latched) -> [cellLatch2]
  [cellLatch1] -> Mux1/1
  [cellLatch2] -> Mux1/2
  [cellLatch3] -> Mux1/3
  [cellLatch4] -> Mux1/4
  [cellLatch5] -> Mux1/5
  [cellLatch6] -> Mux1/6
  [cellLatch7] -> Mux1/7
  [cellLatch8] -> Mux1/8
  [cellLatch9] -> Mux1/9
  [cellLatch10] -> Mux1/10
  [cellLatch11] -> Mux1/11
  [cellLatch12] -> Mux1/12
  [cellLatch13] -> Mux1/13
  [cellLatch14] -> Mux1/14
  [cellLatch15] -> Mux1/15
  [cellLatch16] -> Mux1/16
  [cellLatch17] -> Mux1/17
  [cellLatch18] -> Mux1/18
  [cellLatch19] -> Mux1/19
  [cellLatch20] -> Mux1/20
  [cellLatch21] -> Mux1/21
  Object1/3(objPose) -> [cellPose1]
  Object2/3(objPose) -> [cellPose2]
  [cellPose1] -> Vector Concatenate/1
  [cellPose2] -> Vector Concatenate/2
  [cellPose3] -> Vector Concatenate/3
  Vector Concatenate/1 -> MATLAB Function2/2(cellPoses)
  [cellPose4] -> Vector Concatenate/4
  [gripY] -> Rate Transition/1
  [gripX] -> Rate Transition1/1
  Rate Transition1/1 -> Mux2/1
  Rate Transition/1 -> Mux2/2
  Mux2/1 -> MATLAB Function2/1(robotPose)
  MATLAB Function2/1(cellTarget) -> Delay1/1
  Delay1/1 -> [targetCell]
  [targetCell] -> Object1/4(In4)
  [cellPose5] -> Vector Concatenate/5
  [cellPose6] -> Vector Concatenate/6
  [cellPose7] -> Vector Concatenate/7
  [cellPose8] -> Vector Concatenate/8
  [cellPose9] -> Vector Concatenate/9
  [cellPose10] -> Vector Concatenate/10
  [cellPose11] -> Vector Concatenate/11
  [cellPose12] -> Vector Concatenate/12
  [cellPose13] -> Vector Concatenate/13
  [cellPose14] -> Vector Concatenate/14
  [cellPose15] -> Vector Concatenate/15
  [cellPose16] -> Vector Concatenate/16
  [cellPose17] -> Vector Concatenate/17
  [cellPose18] -> Vector Concatenate/18
  [cellPose19] -> Vector Concatenate/19
  [cellPose20] -> Vector Concatenate/20
  [cellPose21] -> Vector Concatenate/21
  [inuse] -> Object2/3(In3)
  [latch] -> Object2/1(In1)
  [scoreLevel] -> Object2/2(In2)
  [targetCell] -> Object2/4(In4)
  [latch] -> Object3/1(In1)
  [targetCell] -> Object3/4(In4)
  [scoreLevel] -> Object3/2(In2)
  [inuse] -> Object3/3(In3)
  [latch] -> Object4/1(In1)
  [targetCell] -> Object4/4(In4)
  [scoreLevel] -> Object4/2(In2)
  [inuse] -> Object4/3(In3)
  [latch] -> Object5/1(In1)
  [targetCell] -> Object5/4(In4)
  [scoreLevel] -> Object5/2(In2)
  [inuse] -> Object5/3(In3)
  [latch] -> Object6/1(In1)
  [targetCell] -> Object6/4(In4)
  [scoreLevel] -> Object6/2(In2)
  [inuse] -> Object6/3(In3)
  [latch] -> Object7/1(In1)
  [targetCell] -> Object7/4(In4)
  [scoreLevel] -> Object7/2(In2)
  [inuse] -> Object7/3(In3)
  Object3/1(cellType) -> [celltype3]
  Object3/2(latched) -> [cellLatch3]
  Object3/3(objPose) -> [cellPose3]
  Object4/1(cellType) -> [celltype4]
  Object4/2(latched) -> [cellLatch4]
  Object4/3(objPose) -> [cellPose4]
  Object5/3(objPose) -> [cellPose5]
  Object5/2(latched) -> [cellLatch5]
  Object5/1(cellType) -> [celltype5]
  Object6/1(cellType) -> [celltype6]
  Object6/2(latched) -> [cellLatch6]
  Object6/3(objPose) -> [cellPose6]
  Object7/3(objPose) -> [cellPose7]
  Object7/2(latched) -> [cellLatch7]
  Object7/1(cellType) -> [celltype7]
  [scoreLevel] -> Object8/2(In2)
  [latch] -> Object8/1(In1)
  [inuse] -> Object8/3(In3)
  [targetCell] -> Object8/4(In4)
  [inuse] -> Object9/3(In3)
  [latch] -> Object9/1(In1)
  [targetCell] -> Object9/4(In4)
  [scoreLevel] -> Object9/2(In2)
  [inuse] -> Object10/3(In3)
  [latch] -> Object10/1(In1)
  [targetCell] -> Object10/4(In4)
  [scoreLevel] -> Object10/2(In2)
  [inuse] -> Object11/3(In3)
  [latch] -> Object11/1(In1)
  [targetCell] -> Object11/4(In4)
  [scoreLevel] -> Object11/2(In2)
  [inuse] -> Object12/3(In3)
  [latch] -> Object12/1(In1)
  [targetCell] -> Object12/4(In4)
  [scoreLevel] -> Object12/2(In2)
  [inuse] -> Object13/3(In3)
  [latch] -> Object13/1(In1)
  [targetCell] -> Object13/4(In4)
  [scoreLevel] -> Object13/2(In2)
  [inuse] -> Object14/3(In3)
  [latch] -> Object14/1(In1)
  [targetCell] -> Object14/4(In4)
  [scoreLevel] -> Object14/2(In2)
  Object8/3(objPose) -> [cellPose8]
  Object8/1(cellType) -> [celltype8]
  Object8/2(latched) -> [cellLatch8]
  Object9/1(cellType) -> [celltype9]
  Object9/2(latched) -> [cellLatch9]
  Object9/3(objPose) -> [cellPose9]
  Object10/1(cellType) -> [celltype10]
  Object10/2(latched) -> [cellLatch10]
  Object10/3(objPose) -> [cellPose10]
  Object11/3(objPose) -> [cellPose11]
  Object11/1(cellType) -> [celltype11]
  Object11/2(latched) -> [cellLatch11]
  Object12/1(cellType) -> [celltype12]
  Object12/2(latched) -> [cellLatch12]
  Object12/3(objPose) -> [cellPose12]
  Object13/1(cellType) -> [celltype13]
  Object13/2(latched) -> [cellLatch13]
  Object13/3(objPose) -> [cellPose13]
  Object14/1(cellType) -> [celltype14]
  Object14/2(latched) -> [cellLatch14]
  Object14/3(objPose) -> [cellPose14]
  Object18/3(objPose) -> [cellPose18]
  Object21/2(latched) -> [cellLatch21]
  Object19/2(latched) -> [cellLatch19]
  [targetCell] -> Object15/4(In4)
  [scoreLevel] -> Object15/2(In2)
  Object17/2(latched) -> [cellLatch17]
  [latch] -> Object15/1(In1)
  [targetCell] -> Object16/4(In4)
  [inuse] -> Object16/3(In3)
  Object20/2(latched) -> [cellLatch20]
  Object17/3(objPose) -> [cellPose17]
  Object19/3(objPose) -> [cellPose19]
  [targetCell] -> Object21/4(In4)
  Object21/1(cellType) -> [celltype21]
  [latch] -> Object21/1(In1)
  Object15/2(latched) -> [cellLatch15]
  [inuse] -> Object21/3(In3)
  [scoreLevel] -> Object20/2(In2)
  [latch] -> Object16/1(In1)
  Object16/1(cellType) -> [celltype16]
  [inuse] -> Object20/3(In3)
  Object20/1(cellType) -> [celltype20]
  [inuse] -> Object15/3(In3)
  Object15/3(objPose) -> [cellPose15]
  Object19/1(cellType) -> [celltype19]
  Object15/1(cellType) -> [celltype15]
  [targetCell] -> Object20/4(In4)
  [latch] -> Object17/1(In1)
  [scoreLevel] -> Object17/2(In2)
  Object16/3(objPose) -> [cellPose16]
  Object21/3(objPose) -> [cellPose21]
  Object16/2(latched) -> [cellLatch16]
  Object20/3(objPose) -> [cellPose20]
  Object17/1(cellType) -> [celltype17]
  [inuse] -> Object17/3(In3)
  [scoreLevel] -> Object19/2(In2)
  [scoreLevel] -> Object21/2(In2)
  Object18/1(cellType) -> [celltype18]
  [targetCell] -> Object19/4(In4)
  [targetCell] -> Object17/4(In4)
  [scoreLevel] -> Object16/2(In2)
  [inuse] -> Object19/3(In3)
  [scoreLevel] -> Object18/2(In2)
  [targetCell] -> Object18/4(In4)
  Object18/2(latched) -> [cellLatch18]
  [latch] -> Object19/1(In1)
  [latch] -> Object18/1(In1)
  [latch] -> Object20/1(In1)
  [inuse] -> Object18/3(In3)
  Data Type Conversion/1 -> [scoreLevel]
  connections:
  Object1/LConn1 -- Object17/LConn1 -- Object21/LConn1 -- Object20/LConn1 -- Object19/LConn1 -- Object18/LConn1 -- Object16/LConn1 -- Object15/LConn1 -- Object14/LConn1 -- Object13/LConn1 -- Object12/LConn1 -- Object11/LConn1 -- Object10/LConn1 -- Object9/LConn1 -- Object8/LConn1 -- Object7/LConn1 -- Object6/LConn1 -- Object5/LConn1 -- Object4/LConn1 -- RP-Bus/RConn1 -- Object3/LConn1 -- Object2/LConn1

== system AutonomousModel_V3/BEST Robotics 2020 Game (Double-Click)/Compass Sensor ==
  angle : Inport
  Rate Transition : RateTransition  OutPortSampleTime=sensorTs
  Distance : Outport  VectorParamsAs1DForOutWhenUnconnected=off
  wires:
  angle/1 -> Rate Transition/1
  Rate Transition/1 -> Distance/1

== system AutonomousModel_V3/BEST Robotics 2020 Game (Double-Click)/Game Control ==
  Compare To Constant : simulink/Logic and Bit Operations/Compare To Constant  relop=>  const=gameTime + 0.1  OutDataTypeStr=boolean
  Digital Clock : DigitalClock  SampleTime=0.1
  Stop Simulation : Stop
  To Workspace : ToWorkspace  VariableName=GameResults  SampleTime=-1
      settings: MaxDataPoints=1
  Vector Concatenate : Concatenate  NumInputs=24  Mode=Multidimensional array
  wires:
  Compare To Constant/1 -> Stop Simulation/1
  Digital Clock/1 -> Compare To Constant/1
  Vector Concatenate/1 -> To Workspace/1
  [objInfo1] -> Vector Concatenate/1
  [objInfo2] -> Vector Concatenate/2
  [objInfo3] -> Vector Concatenate/3
  [objInfo4] -> Vector Concatenate/4
  [objInfo5] -> Vector Concatenate/5
  [objInfo6] -> Vector Concatenate/6
  [objInfo7] -> Vector Concatenate/7
  [objInfo8] -> Vector Concatenate/8
  [objInfo9] -> Vector Concatenate/9
  [objInfo10] -> Vector Concatenate/10
  [objInfo11] -> Vector Concatenate/11
  [objInfo12] -> Vector Concatenate/12
  [objInfo13] -> Vector Concatenate/13
  [objInfo14] -> Vector Concatenate/14
  [objInfo15] -> Vector Concatenate/15
  [objInfo16] -> Vector Concatenate/16
  [objInfo17] -> Vector Concatenate/17
  [objInfo18] -> Vector Concatenate/18
  [objInfo19] -> Vector Concatenate/19
  [objInfo20] -> Vector Concatenate/20
  [objInfo21] -> Vector Concatenate/21
  [vacInfo1] -> Vector Concatenate/22
  [vacInfo2] -> Vector Concatenate/23
  [vacInfo3] -> Vector Concatenate/24

== system AutonomousModel_V3/BEST Robotics 2020 Game (Double-Click)/Left Encoder1 ==
  In1 : Inport
  Input : Inport  Port=2
  Abs : Abs  ZeroCross=off
  Constant : Constant  Value=detectDir
  Gain2 : Gain  Gain=180/pi
  Gain3 : Gain  Gain=ticks/360
  Integrator : Integrator  ExternalReset=rising
  Rate Transition : RateTransition  OutPortSampleTime=sensorTs
  Rounding Function : Rounding  Operator=ceil
  Switch : Switch  Criteria=u2 ~= 0
  Out1 : Outport  VectorParamsAs1DForOutWhenUnconnected=off
  wires:
  Rate Transition/1 -> Out1/1
  Rounding Function/1 -> Rate Transition/1
  Gain3/1 -> Rounding Function/1
  Gain2/1 -> Integrator/1
  Integrator/1 -> Gain3/1
  Input/1 -> Integrator/2
  Switch/1 -> Gain2/1
  In1/1 -> Abs/1, Switch/1
  Constant/1 -> Switch/2
  Abs/1 -> Switch/3

== system AutonomousModel_V3/BEST Robotics 2020 Game (Double-Click)/Right Encoder1 ==
  In1 : Inport
  Input : Inport  Port=2
  Abs : Abs  ZeroCross=off
  Constant : Constant  Value=detectDir
  Gain2 : Gain  Gain=180/pi
  Gain3 : Gain  Gain=ticks/360
  Integrator : Integrator  ExternalReset=rising
  Rate Transition : RateTransition  OutPortSampleTime=sensorTs
  Rounding Function : Rounding  Operator=ceil
  Switch : Switch  Criteria=u2 ~= 0
  Out1 : Outport  VectorParamsAs1DForOutWhenUnconnected=off
  wires:
  Abs/1 -> Switch/3
  Constant/1 -> Switch/2
  In1/1 -> Switch/1, Abs/1
  Switch/1 -> Gain2/1
  Input/1 -> Integrator/2
  Integrator/1 -> Gain3/1
  Gain2/1 -> Integrator/1
  Gain3/1 -> Rounding Function/1
  Rounding Function/1 -> Rate Transition/1
  Rate Transition/1 -> Out1/1

== system AutonomousModel_V3/BEST Robotics 2020 Game (Double-Click)/Vaccines ==
  "ScoreLevel " : Inport
  Drop : Inport  Port=2
  Data Type Conversion1 : DataTypeConversion
  Demux : Demux  Outputs=3
  Vaccine : Subsystem  mask(RP Rectangle-Disc obstacle){}
      mask help: This block introduces a rectangle obstacle to the virtual environment. The obstacle dynamics include exerting the necessary contact forces with the robots as well as detectability by the ultrasonic sensor when used in a MathWorks provided virtual environment.
  Vaccine1 : Subsystem  mask(RP Rectangle-Disc obstacle){}
      mask help: This block introduces a rectangle obstacle to the virtual environment. The obstacle dynamics include exerting the necessary contact forces with the robots as well as detectability by the ultrasonic sensor when used in a MathWorks provided virtual environment.
  Vaccine2 : Subsystem  mask(RP Rectangle-Disc obstacle){}
      mask help: This block introduces a rectangle obstacle to the virtual environment. The obstacle dynamics include exerting the necessary contact forces with the robots as well as detectability by the ultrasonic sensor when used in a MathWorks provided virtual environment.
  RP-Bus : PMIOPort  Side=Left
  wires:
  Drop/1 -> Data Type Conversion1/1
  Data Type Conversion1/1 -> Demux/1
  Demux/1 -> Vaccine/1(Drop)
  "ScoreLevel "/1 -> Vaccine2/2(ScoreLevel), Vaccine1/2(ScoreLevel), Vaccine/2(ScoreLevel)
  Demux/2 -> Vaccine1/1(Drop)
  Demux/3 -> Vaccine2/1(Drop)
  connections:
  Vaccine/LConn1 -- RP-Bus/RConn1 -- Vaccine2/LConn1 -- Vaccine1/LConn1
